simulink model "PMSM_Sensorless_MARS_idq_prime"  (R2024b)
settings: Solver=FixedStepAuto  StartTime=0.0  StopTime=0.5  FixedStep=1e-6  RelTol=1e-3
model workspace (MAT data in the model file):
  B = 0
  Current_Filter_On = 0
  F = 10000
  J = 5.8e-05
  Ls = 0.0005125
  MRAS_Ki = 0.3
  MRAS_Kp = 0.7
  PLL_Ki = 800
  PLL_Kp = 1000
  Pn = 5
  Rs = 0.1445
  T_deadband = 0
  Ts = 5e-05
  Vdc = 60
  id_ki = 289
  id_kp = 1.025
  iq_ki = 289
  iq_kp = 1.025
  k = 150
  l_asmo = 2000
  psi_f = 0.0113
  speed_ki = 10
  speed_kp = 0.05
  w_c = 8000
undefined symbols (not defined in the file): sigbuilder_block
libraries: dspfdesign x5, slpidlib x4, simulink x2, spsDCVoltageSourceLib x1, spsOnDelayLib x1, spsGroundLib x1, dsparch4 x1, spsPermanentMagnetSynchronousMachineLib x1, spsThreePhaseVIMeasurementLib x1, spsTwoLevelConverterLib x1, spspowerguiLib x1
(part 2 of 2)

== system PMSM_Sensorless_MARS_idq_prime/Filter/LowpassFilter/Lowpass filter3 ==
  K : Inport
  u(t) : Inport  Port=2
  Add : Sum
  Delay : Delay  DelayLength=1
  Product : Product
  Subtract : Sum  Inputs=+-
  Ic : Outport
  wires:
  Add/1 -> Ic/1, Delay/1
  Product/1 -> Add/1
  Subtract/1 -> Product/2
  Delay/1 -> Subtract/2, Add/2
  K/1 -> Product/1
  u(t)/1 -> Subtract/1

== matlab function PMSM_Sensorless_MARS_idq_prime/MATLAB Function ==
  data: angle input; theta_2pi output
function theta_2pi = Angle_Conv(angle)

theta_2pi=mod(angle,2*pi);

== matlab function PMSM_Sensorless_MARS_idq_prime/PLL1/MATLAB Function1 ==
  data: angle input; theta_2pi output
function theta_2pi = Angle_Conv(angle)

theta_2pi=mod(angle,2*pi);

== matlab function PMSM_Sensorless_MARS_idq_prime/FOC//SVPWM Algorithm/CCR_Generator ==
  data: CNT input; Tcmp1 input; Tcmp2 input; Tcmp3 input; CH1 output; CH1N output; CH2 output; CH2N output; CH3 output; CH3N output
function[CH1,CH1N,CH2,CH2N,CH3,CH3N] = CCR_Generator(CNT,Tcmp1, Tcmp2, Tcmp3)

if (CNT<Tcmp1)
    CH1=0;
    CH1N=1;
else
    CH1=1;
    CH1N=0;
end
if (CNT<Tcmp2)
    CH2=0;
    CH2N=1;
else
    CH2=1;
    CH2N=0;
end
if (CNT<Tcmp3)
    CH3=0;
    CH3N=1;
else
    CH3=1;
    CH3N=0;
end
end

== matlab function PMSM_Sensorless_MARS_idq_prime/FOC//SVPWM Algorithm/SVPWM/OverModulationHandle ==
  data: T1_RAW input; T2_RAW input; T1 output; T2 output; Ts input
function [T1,T2] = OverModulationHandle(T1_RAW, T2_RAW, Ts)
if((T1_RAW+T2_RAW)>Ts)
    T1=T1_RAW/(T1_RAW+T2_RAW)*Ts;
    T2=T2_RAW/(T1_RAW+T2_RAW)*Ts;
else
    T1=T1_RAW;
    T2=T2_RAW;
end
end

== matlab function PMSM_Sensorless_MARS_idq_prime/PLL/MATLAB Function1 ==
  data: angle input; theta_2pi output
function theta_2pi = Angle_Conv(angle)

theta_2pi=mod(angle,2*pi);

== matlab function PMSM_Sensorless_MARS_idq_prime/MRAS/可调模型 ==
  data: id_prime_hat input; id_dot_prime_hat output; iq_prime_hat input; Rs input; Ls input; iq_dot_prime_hat output; we_hat input; ud_prime input; uq_prime input
function [id_dot_prime_hat,iq_dot_prime_hat] = fcn(id_prime_hat,iq_prime_hat,Rs,Ls,we_hat,ud_prime,uq_prime)

id_dot_prime_hat = -Rs/Ls*id_prime_hat+we_hat*iq_prime_hat+1/Ls*ud_prime;
iq_dot_prime_hat = -Rs/Ls*iq_prime_hat-we_hat*id_prime_hat+1/Ls*uq_prime;

== matlab function PMSM_Sensorless_MARS_idq_prime/MRAS/MATLAB Function2 ==
  data: angle input; theta_2pi output
function theta_2pi = Angle_Conv(angle)

theta_2pi=mod(angle,2*pi);
